simulink model "ctdsm_3OrderFF"  (R2025b)
settings: Solver=VariableStepAuto  StartTime=0.0  StopTime=1  RelTol=1e-6
undefined symbols (not defined in the file or in its folder): aff, fs
libraries: msbAdcFoundation x1, dspquant2 x1
settings Model: Creator=The MathWorks, Inc.  LastModifiedBy=The MathWorks, Inc.
settings RTWCC: LargeConstantGeneration=WriteOnlyDNNConstantsToDataFiles

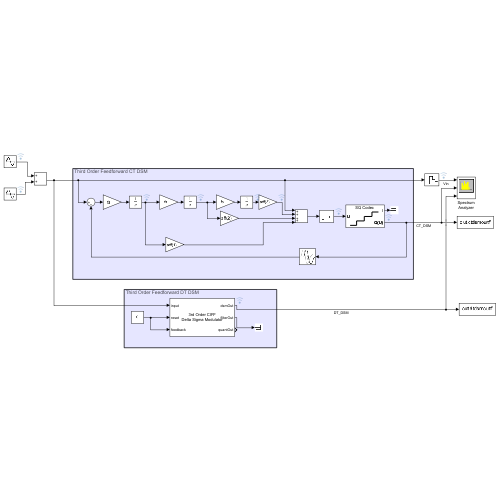
[thumbnail: Simulink's stored preview of the top-level diagram]
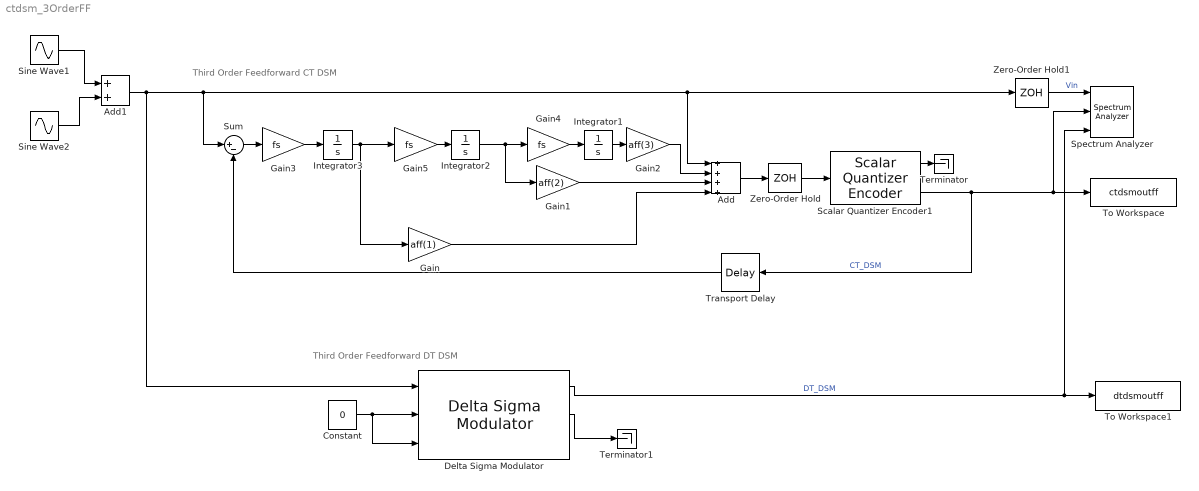
== system ctdsm_3OrderFF ==
  note: Third Order Feedforward CT DSM
  note: Third Order Feedforward DT DSM
  Add : Sum  Inputs=++++
  Add1 : Sum
  Constant : Constant  Value=0
  Delta Sigma Modulator : msbAdcFoundation/Delta Sigma Modulator  dsmArchitecture=CIFF  dsmOrder=3rd order  BandWidth=1000  OSR=64  SamplingFrequency=128000  NumberLevels=16  QuantizerOutput=-15:2:15  BoundaryPoints=[-8:1:8]  EnableDynamicRangeScaling=off  EnableCustomCoeff=off  a=[0.6666 0.2038 0.0270]  g=[0.0000]  b=[1.0000 0.0000 0.0000 1.0000]  c=[1.0000 1.0000 1.0000]  OLgain=Inf  EnableNoise=off  thermalNoiseValue=200e-6  thermalNoiseUnit=Vrms  refResistance=50  wNoiseGain=0.0002  fcorner=1000  pNoiseGain=5e-06  ntfOptim=0: Unoptimized  passbandType=Lowpass  centerFrequency=0  EnableCustomHinf=off  Hinf=1.4  NTFflag=on  PZflag=off  STFflag=off  SNRflag=off  AppendFlag=off  ExportFlag=off
      link override Delta Sigma Modulator: LabelModeActiveChoice=3CIFF
      link override Noise: LabelModeActiveChoice=noNoise
  Gain : Gain  Gain=aff(1)
  Gain1 : Gain  Gain=aff(2)
  Gain2 : Gain  Gain=aff(3)
  Gain3 : Gain  Gain=fs
  Gain4 : Gain  Gain=fs
  Gain5 : Gain  Gain=fs
  Integrator1 : Integrator
  Integrator2 : Integrator
  Integrator3 : Integrator
  Scalar Quantizer Encoder1 : dspquant2/Scalar Quantizer Encoder  paramSrc=Specify via dialog  partType=Bounded  BBoundary=[-15:2:17]  UBoundary=[2:9]  SearchMethod=Linear  tieBreakRule=Choose the lower index  outQU=on  outQError=off  codebook=[-15:2:15]  outStatus=off  invalidin=Clip  idtype=int8  roundingMode=Floor  overflowMode=off
  Sine Wave1 : Sin  Amplitude=0.8*15  Frequency=2*pi*500  SampleTime=0
  Sine Wave2 : Sin  Amplitude=0.1815  Frequency=2*pi*0.99*fs  Phase=pi  SampleTime=0
  Spectrum Analyzer : SpectrumAnalyzer  NumInputPorts=3  WindowPosition=[44.000000,38.000000,1224.000000,711.000000,]  ScopeFrameLocation=window  PlotAsTwoSidedSpectrum=off  FrequencyScale=Log  Span=50  CenterFrequency=25  StartFrequency=0  StopFrequency=50  YLimits=[-107.12195564,65.86960616]  ColorLimits=[-20 80]  ShowLegend=on  AllowFFTLengthLessThanSamplesPerUpdate=on  DefaultConfigurationName=spbscopes.SpectrumAnalyzerBlockCfg  IsFrequencyInputMode=0  FrequencyVectorPort=0  FrequencyVectorFromPort=0  FrequencyInputRBWPort=0  FrequencyInputRBWFromPort=0
  Sum : Sum  Inputs=|+-
  Terminator : Terminator
  Terminator1 : Terminator
  To Workspace : ToWorkspace  VariableName=ctdsmoutff  SampleTime=-1
      settings: MaxDataPoints=fs
  To Workspace1 : ToWorkspace  VariableName=dtdsmoutff  SampleTime=-1
      settings: MaxDataPoints=fs
  Transport Delay : TransportDelay  DelayTime=0.1/fs
  Zero-Order Hold : ZeroOrderHold  SampleTime=1/fs
  Zero-Order Hold1 : ZeroOrderHold  SampleTime=1/fs
  wires:
  Scalar Quantizer Encoder1/1 -> Terminator/1
  Zero-Order Hold/1 -> Scalar Quantizer Encoder1/1
  Add/1 -> Zero-Order Hold/1
  Integrator2/1 -> Gain4/1, Gain1/1
  Scalar Quantizer Encoder1/2 -> To Workspace/1, Spectrum Analyzer/2, Transport Delay/1  "CT_DSM"
  Integrator1/1 -> Gain2/1
  Integrator3/1 -> Gain5/1, Gain/1
  Sum/1 -> Gain3/1
  Add1/1 -> Delta Sigma Modulator/1, Sum/1, Zero-Order Hold1/1, Add/1
  Transport Delay/1 -> Sum/2
  Gain/1 -> Add/4
  Gain1/1 -> Add/3
  Gain2/1 -> Add/2
  Gain4/1 -> Integrator1/1
  Gain5/1 -> Integrator2/1
  Sine Wave1/1 -> Add1/1
  Sine Wave2/1 -> Add1/2
  Zero-Order Hold1/1 -> Spectrum Analyzer/1  "Vin"
  Gain3/1 -> Integrator3/1
  Delta Sigma Modulator/2 -> Terminator1/1
  Constant/1 -> Delta Sigma Modulator/3, Delta Sigma Modulator/2
  Delta Sigma Modulator/1 -> Spectrum Analyzer/3, To Workspace1/1  "DT_DSM"
